simulink model "P2_simulink"  (R2017a)
settings: Solver=ode45  StartTime=0.0  StopTime=10.0  RelTol=1e-3  EnableMultiTasking=on
values from neighbouring files (symbols this model uses):
  b = 0.5    [P2_comparacion.m]    (also in P2_script_lineal.m; P2_script_no_lineal.m; mrm.m = 8)
  g = 9.8    [P2_comparacion.m]    (also in P2_script_lineal.m; P2_script_no_lineal.m)
  K = 2    [P2_comparacion.m]    (also in P2_script_lineal.m; P2_script_no_lineal.m; mrm.m = 273)
  L = 0.01    [P2_comparacion.m]    (also in P2_script_lineal.m; P2_script_no_lineal.m)
  M = 0.2    [P2_comparacion.m]    (also in P2_script_lineal.m; P2_script_no_lineal.m)
  R = 20    [P2_comparacion.m]    (also in P2_script_lineal.m; P2_script_no_lineal.m)
settings Model: Creator=Administrador  LastModifiedBy=joaqu
settings DataIOCC: LimitDataPoints=on  SaveFormat=Array
settings OptimizationCC: LifeSpan=inf
settings DebuggingCC: SolverPrmCheckMsg=warning  SFUnexpectedBacktrackingDiag=warning  SFNoUnconditionalDefaultTransitionDiag=warning  SFExecutionAtInitializationDiag=none
settings HardwareCC: ProdBitPerPointer=32  ProdBitPerSizeT=32  ProdBitPerPtrDiffT=32  ProdLargestAtomicFloat=None  ProdIntDivRoundTo=Undefined  ProdEndianess=Unspecified  ProdWordSize=32  ProdHWDeviceType=32-bit Generic
settings ModelReferenceCC: PropagateSignalLabelsOutOfModel=off
settings GRTTargetCC: TargetLangStandard=C89/C90 (ANSI)  GeneratePreprocessorConditionals=Disable all
settings ConfigComp: CovMetricSettings=dw  CovHtmlReporting=on  CovSaveCumulativeToWorkspaceVar=on  CovSaveSingleToWorkspaceVar=on  CovExternalEMLEnable=off  CovSFcnEnable=off

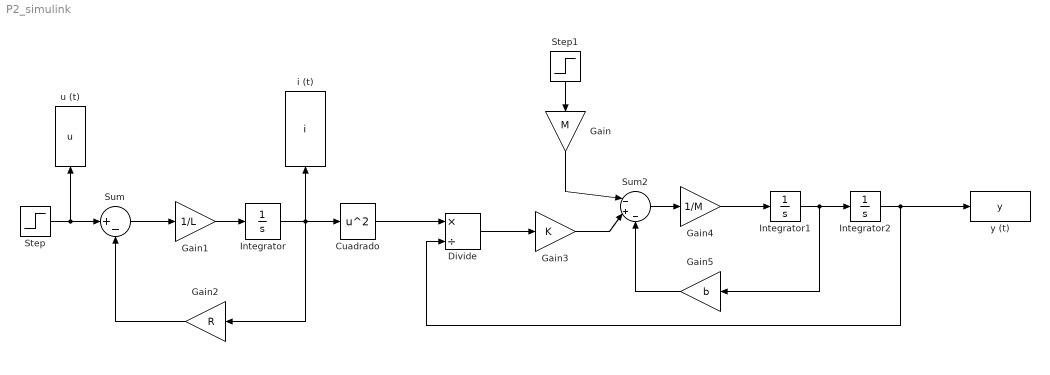
== system P2_simulink ==
  " i (t)" : ToWorkspace  VariableName=i  SaveFormat=Timeseries  SampleTime=-1
  " u (t)" : ToWorkspace  VariableName=u  SaveFormat=Timeseries  SampleTime=-1
  Cuadrado : Math  Operator=square  SaturateOnIntegerOverflow=on
  Divide : Product  Inputs=*/
  Gain : Gain  Gain=M
  Gain1 : Gain  Gain=1/L
  Gain2 : Gain  Gain=R
  Gain3 : Gain  Gain=K
  Gain4 : Gain  Gain=1/M
  Gain5 : Gain  Gain=b
  Integrator : Integrator  InitialCondition=0.5
  Integrator1 : Integrator
  Integrator2 : Integrator  InitialCondition=0.2551
  Step : Step  Time=0  Before=10  After=10.2  SampleTime=0
  Step1 : Step  Time=0  After=g  SampleTime=0
  Sum : Sum  Inputs=|+-
  Sum2 : Sum  Inputs=|-+-
  y (t) : ToWorkspace  VariableName=y  SaveFormat=Timeseries  SampleTime=-1
  wires:
  Sum/1 -> Gain1/1
  Gain1/1 -> Integrator/1
  Integrator/1 -> " i (t)"/1, Cuadrado/1, Gain2/1
  Gain2/1 -> Sum/2
  Integrator1/1 -> Gain5/1, Integrator2/1
  Integrator2/1 -> y (t)/1, Divide/2
  Gain4/1 -> Integrator1/1
  Step/1 -> " u (t)"/1, Sum/1
  Step1/1 -> Gain/1
  Gain/1 -> Sum2/1
  Gain5/1 -> Sum2/3
  Sum2/1 -> Gain4/1
  Cuadrado/1 -> Divide/1
  Divide/1 -> Gain3/1
  Gain3/1 -> Sum2/2
